simulink model "BdotControl_STAB_SUN_GRAV"  (R2019b)
settings: Solver=FixedStepAuto  StartTime=0.0  StopTime=dm.init.duration  FixedStep=fsw.init.dt  RelTol=1e-3
InitFcn:
  | clearvars;
  | % init_param_6U;
  |  init_param_6U_AW;
  | % init_param_FS_ISSorbit;
undefined symbols (not defined in the file or in its folder): dm, Earth, fsw, K_bdot, K_theta, WGS84
libraries: vrlib x4, dspmathops x3, aerolibtransform2 x2, simulink x1, aerolibgravity2 x1
settings Model: SimulationMode=accelerator  Creator=Jack-AOCS  LastModifiedBy=AndrewWang
settings DataIOCC: ReturnWorkspaceOutputs=off
settings DebuggingCC: ArithmeticOperatorsInVariantConditions=warning
settings SFSimCC: SimUseLocalCustomCode=off  CustomCodeUndefinedFunction=UseInterfaceOnly
settings RTWCC: RTWUseLocalCustomCode=off

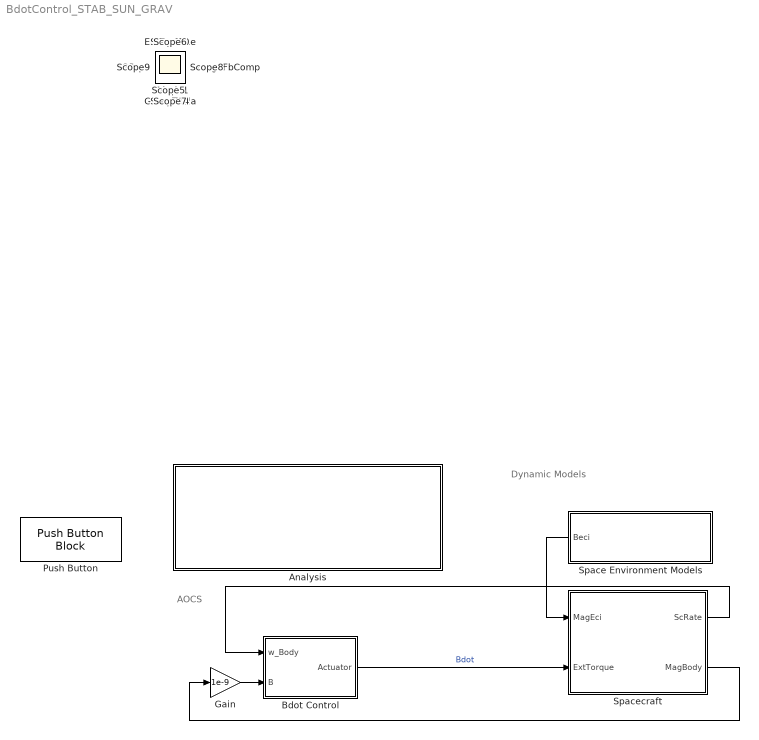
== system BdotControl_STAB_SUN_GRAV ==
  note: AOCS
  note: Dynamic Models
  Analysis : Subsystem
  Bdot Control : Subsystem
  Gain : Gain  Gain=1e-9
  Push Button : PushButtonBlock
  Space Environment Models : Subsystem
  Spacecraft : Subsystem
  BdotMc : Scope
  ExtTvsRate : Scope
  GaussTesla : Scope
  OmegaFbComp : Scope
  Rate : Scope
  Scope{,1..2,4..10,14} (11 alike) : Scope
  wires:
  Spacecraft/2(MagBody) -> Gain/1
  Space Environment Models/1(Beci) -> Spacecraft/1(MagEci)
  Bdot Control/1(Actuator) -> Spacecraft/2(ExtTorque)  "Bdot"
  Gain/1 -> Bdot Control/2(B)
  Spacecraft/1(ScRate) -> Bdot Control/1(w_Body)

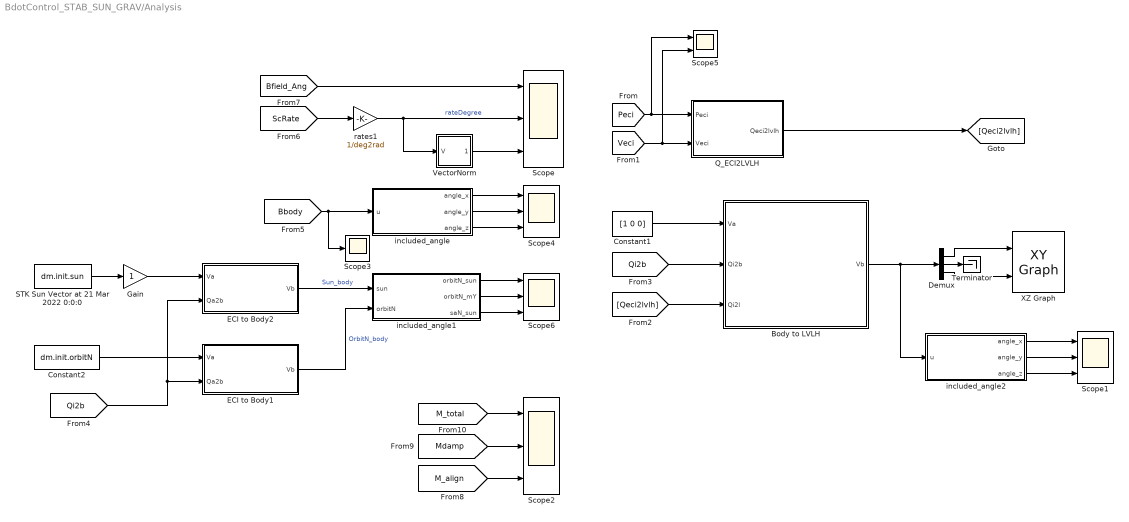
== system BdotControl_STAB_SUN_GRAV/Analysis ==
  Body to LVLH : MATLAB Function  TreatAsAtomicUnit=on
  Constant1 : Constant  Value=[1 0 0]
  Constant2 : Constant  Value=dm.init.orbitN
  Demux : Demux  Outputs=3
  ECI to Body1 : MATLAB Function  TreatAsAtomicUnit=on
  ECI to Body2 : MATLAB Function  TreatAsAtomicUnit=on
  Gain : Gain
  Q_ECI2LVLH : MATLAB Function  TreatAsAtomicUnit=on
  "STK Sun Vector at 21 Mar 2022 0:0:0 " : Constant  Value=dm.init.sun
  Scope{,1..2,4,6} (5 alike) : Scope  NumInputPorts=3
  Scope3 : Scope
  Scope5 : Scope  NumInputPorts=2
  Terminator : Terminator
  VectorNorm : Subsystem
  XZ Graph : simulink/Sinks/XY Graph  xmin=-1  xmax=1  ymin=-1  ymax=1  st=-1
  included_angle : MATLAB Function  TreatAsAtomicUnit=on
  included_angle1 : MATLAB Function  TreatAsAtomicUnit=on
  included_angle2 : MATLAB Function  TreatAsAtomicUnit=on
  rates1 : Gain  Gain=1/deg2rad
  wires:
  Q_ECI2LVLH/1(Qeci2lvlh) -> [Qeci2lvlh]
  [Peci] -> Scope5/1, Q_ECI2LVLH/1(Peci)
  Demux/1 -> XZ Graph/1
  Body to LVLH/1(Vb) -> included_angle2/1(u), Demux/1
  Constant1/1 -> Body to LVLH/1(Va)
  Demux/3 -> XZ Graph/2
  Demux/2 -> Terminator/1
  [Qeci2lvlh] -> Body to LVLH/3(Qi2l)
  [Qi2b] -> Body to LVLH/2(Qi2b)
  ECI to Body1/1(Vb) -> included_angle1/2(orbitN)  "OrbitN_body"
  "STK Sun Vector at 21 Mar 2022 0:0:0 "/1 -> Gain/1
  Gain/1 -> ECI to Body2/1(Va)
  ECI to Body2/1(Vb) -> included_angle1/1(sun)  "Sun_body"
  [Qi2b] -> ECI to Body2/2(Qa2b), ECI to Body1/2(Qa2b)
  Constant2/1 -> ECI to Body1/1(Va)
  included_angle1/2(orbitN_mY) -> Scope6/2
  included_angle1/3(saN_sun) -> Scope6/3
  included_angle1/1(orbitN_sun) -> Scope6/1
  included_angle/3(angle_z) -> Scope4/3
  included_angle/2(angle_y) -> Scope4/2
  included_angle/1(angle_x) -> Scope4/1
  [Bbody] -> Scope3/1, included_angle/1(u)
  VectorNorm/1(normV) -> Scope/3
  rates1/1 -> VectorNorm/1(V), Scope/2  "rateDegree"
  [ScRate] -> rates1/1
  included_angle2/1(angle_x) -> Scope1/1
  included_angle2/2(angle_y) -> Scope1/2
  included_angle2/3(angle_z) -> Scope1/3
  [M_total] -> Scope2/1
  [Mdamp] -> Scope2/2
  [M_align] -> Scope2/3
  [Bfield_Ang] -> Scope/1
  [Veci] -> Q_ECI2LVLH/2(Veci), Scope5/2

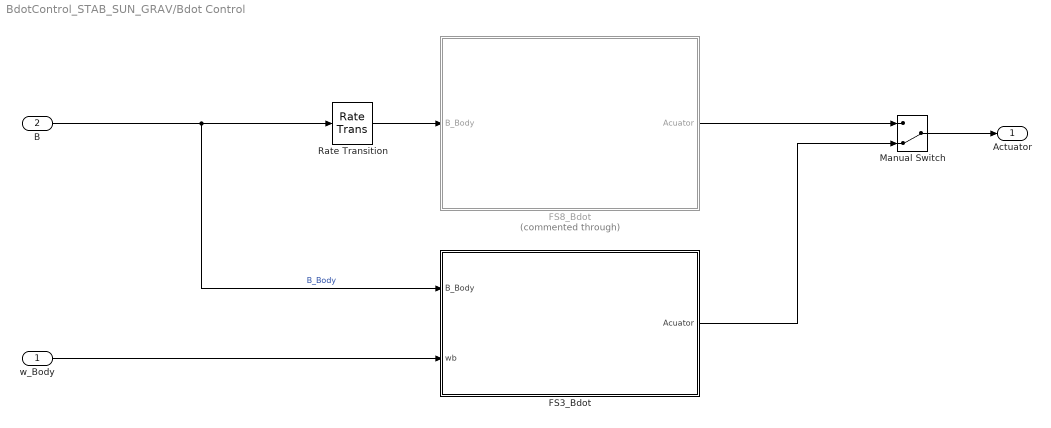
== system BdotControl_STAB_SUN_GRAV/Bdot Control ==
  w_Body : Inport
  B : Inport  Port=2
  FS3_Bdot : Subsystem
  FS8_Bdot : Subsystem  Commented=through
  Manual Switch : ManualSwitch  CurrentSetting=0
  Rate Transition : RateTransition  OutPortSampleTime=fsw.init_FS.dt
  Actuator : Outport  VectorParamsAs1DForOutWhenUnconnected=off
  wires:
  B/1 -> FS3_Bdot/1(B_Body), Rate Transition/1  "B_Body"
  Manual Switch/1 -> Actuator/1
  FS8_Bdot/1(Acuator) -> Manual Switch/1
  FS3_Bdot/1(Acuator) -> Manual Switch/2
  w_Body/1 -> FS3_Bdot/2(wb)
  Rate Transition/1 -> FS8_Bdot/1(B_Body)

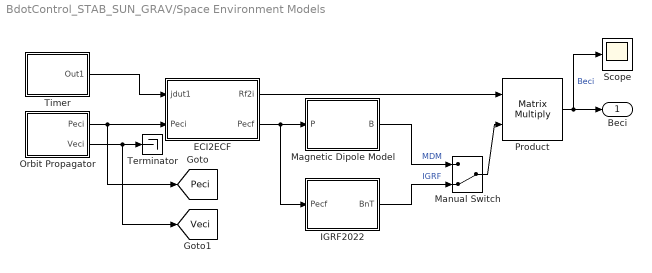
== system BdotControl_STAB_SUN_GRAV/Space Environment Models ==
  ECI2ECF : MATLAB Function  TreatAsAtomicUnit=on
  IGRF2022 : Subsystem
  Magnetic Dipole Model : MATLAB Function  TreatAsAtomicUnit=on
  Manual Switch : ManualSwitch  CurrentSetting=0
  "Orbit Propagator " : Subsystem
  Product : Product  Multiplication=Matrix(*)
  Scope : Scope
  Terminator : Terminator
  Timer : Subsystem
  Beci : Outport  VectorParamsAs1DForOutWhenUnconnected=off
  tag scope: Peci=global, Veci=global
  wires:
  ECI2ECF/1(Rf2i) -> Product/1
  Product/1 -> Scope/1, Beci/1  "Beci"
  "Orbit Propagator "/1(Peci) -> ECI2ECF/2(Peci), [Peci]
  "Orbit Propagator "/2(Veci) -> Terminator/1, [Veci]
  Timer/1(Out1) -> ECI2ECF/1(jdut1)
  ECI2ECF/2(Pecf) -> IGRF2022/1(Pecf), Magnetic Dipole Model/1(P)
  Magnetic Dipole Model/1(B) -> Manual Switch/1  "MDM"
  IGRF2022/1(BnT) -> Manual Switch/2  "IGRF"
  Manual Switch/1 -> Product/2

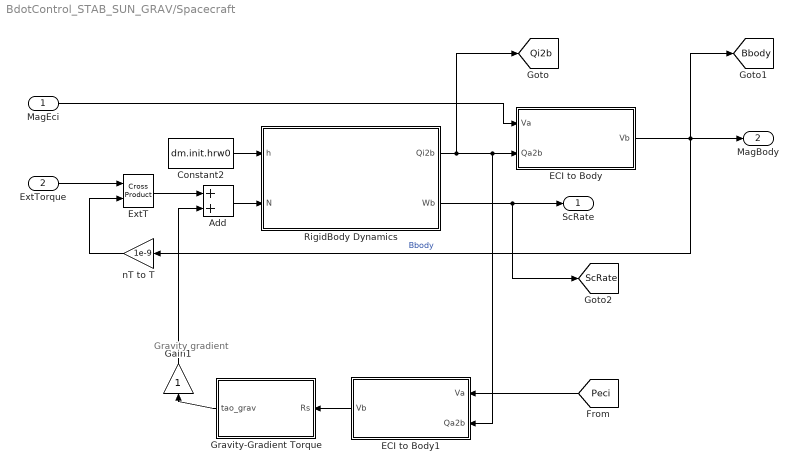
== system BdotControl_STAB_SUN_GRAV/Spacecraft ==
  note: Gravity gradient
  MagEci : Inport
  ExtTorque : Inport  Port=2
  Add : Sum
  Constant2 : Constant  Value=dm.init.hrw0
  ECI to Body : MATLAB Function  TreatAsAtomicUnit=on
  ECI to Body1 : MATLAB Function  TreatAsAtomicUnit=on
  ExtT : vrlib/Utilities/Cross Product
      settings: SourceProductBaseCode=VR
  Gain1 : Gain
  Gravity-Gradient Torque : MATLAB Function  TreatAsAtomicUnit=on
  RigidBody Dynamics : Subsystem
  nT to T : Gain  Gain=1e-9
  ScRate : Outport  VectorParamsAs1DForOutWhenUnconnected=off
  MagBody : Outport  Port=2  VectorParamsAs1DForOutWhenUnconnected=off
  tag scope: Bbody=global, Qi2b=global, ScRate=global
  wires:
  ECI to Body/1(Vb) -> [Bbody], MagBody/1, nT to T/1  "Bbody"
  RigidBody Dynamics/2(Wb) -> [ScRate], ScRate/1
  MagEci/1 -> ECI to Body/1(Va)
  RigidBody Dynamics/1(Qi2b) -> [Qi2b], ECI to Body1/2(Qa2b), ECI to Body/2(Qa2b)
  Constant2/1 -> RigidBody Dynamics/1(h)
  ExtTorque/1 -> ExtT/1
  nT to T/1 -> ExtT/2
  ExtT/1 -> Add/1
  Add/1 -> RigidBody Dynamics/2(N)
  Gravity-Gradient Torque/1(tao_grav) -> Gain1/1
  [Peci] -> ECI to Body1/1(Va)
  ECI to Body1/1(Vb) -> Gravity-Gradient Torque/1(Rs)
  Gain1/1 -> Add/2

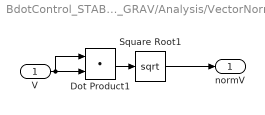
== system BdotControl_STAB_SUN_GRAV/Analysis/VectorNorm ==
  V : Inport
  Dot Product1 : DotProduct  InputSameDT=on  OutDataTypeStr=Inherit: Inherit via internal rule
  Square Root1 : Sqrt  SaturateOnIntegerOverflow=on
  normV : Outport
  wires:
  Dot Product1/1 -> Square Root1/1
  V/1 -> Dot Product1/1, Dot Product1/2
  Square Root1/1 -> normV/1

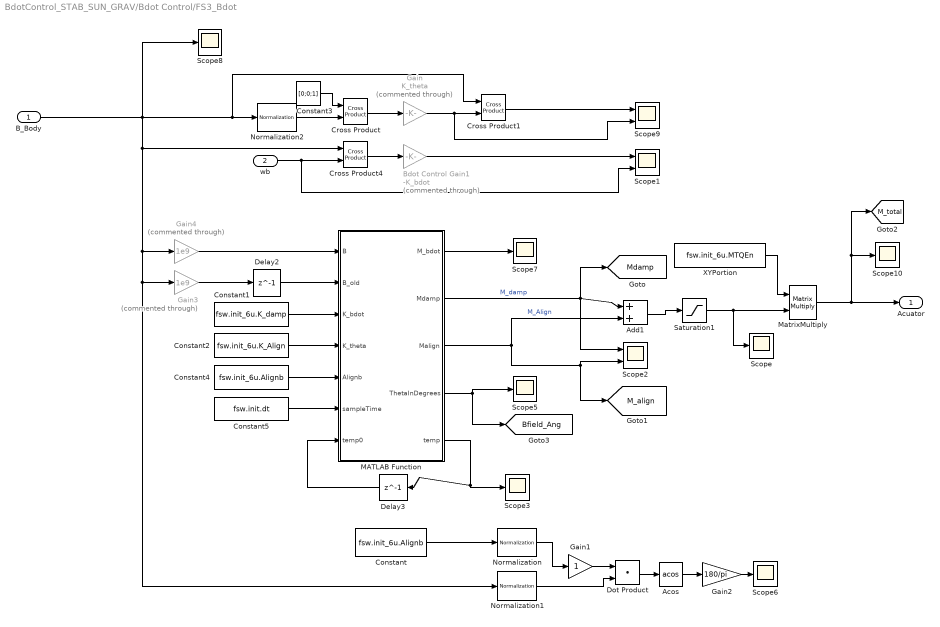
== system BdotControl_STAB_SUN_GRAV/Bdot Control/FS3_Bdot ==
  B_Body : Inport
  wb : Inport  Port=2
  Acos : Trigonometry  Operator=acos
  Add1 : Sum
  Bdot Control Gain1 : Gain  Commented=through  Gain=-K_bdot
  Constant : Constant  Value=fsw.init_6u.Alignb
  Constant1 : Constant  Value=fsw.init_6u.K_damp
  Constant2 : Constant  Value=fsw.init_6u.K_Align
  Constant3 : Constant  Value=[0;0;1]
  Constant4 : Constant  Value=fsw.init_6u.Alignb
  Constant5 : Constant  Value=fsw.init.dt
  Cross Product : vrlib/Utilities/Cross Product
      settings: SourceProductName=Simulink
  Cross Product1 : vrlib/Utilities/Cross Product
      settings: SourceProductName=Simulink
  Cross Product4 : vrlib/Utilities/Cross Product
      settings: SourceProductName=Simulink
  Delay2 : Delay  DelayLength=1  InitialCondition=[0;0;0]
  Delay3 : Delay  DelayLength=1  InitialCondition=[0;0;0]
  Dot Product : DotProduct  InputSameDT=on  OutDataTypeStr=Inherit: Inherit via internal rule
  Gain : Gain  Commented=through  Gain=K_theta
  Gain1 : Gain
  Gain2 : Gain  Gain=180/pi
  Gain3 : Gain  Commented=through  Gain=1e9
  Gain4 : Gain  Commented=through  Gain=1e9
  MATLAB Function : MATLAB Function  TreatAsAtomicUnit=on
  MatrixMultiply : Product  Multiplication=Matrix(*)
  Normalization : dspmathops/Normalization  NormType=2-norm  Bias=1e-10  NormOver=Each column  Dimension=1  roundingMode=Floor  overflowMode=off  accumDataTypeStr=Inherit: Same as product output  accumLastDataTypeStr=Inherit: Same as product output  outputDataTypeStr=Inherit: Same as product output  outputMin=[]  outputMax=[]  outputLastDataTypeStr=Inherit: Same as product output
      settings: SourceProductName=DSP System Toolbox
  Normalization1 : dspmathops/Normalization  NormType=2-norm  Bias=1e-10  NormOver=Each column  Dimension=1  roundingMode=Floor  overflowMode=off  accumDataTypeStr=Inherit: Same as product output  accumLastDataTypeStr=Inherit: Same as product output  outputDataTypeStr=Inherit: Same as product output  outputMin=[]  outputMax=[]  outputLastDataTypeStr=Inherit: Same as product output
      settings: SourceProductName=DSP System Toolbox
  Normalization2 : dspmathops/Normalization  NormType=Squared 2-norm  Bias=1e-10  NormOver=Each column  Dimension=1  roundingMode=Floor  overflowMode=off  accumDataTypeStr=Inherit: Same as product output  accumLastDataTypeStr=Inherit: Same as product output  outputDataTypeStr=Inherit: Same as product output  outputMin=[]  outputMax=[]  outputLastDataTypeStr=Inherit: Same as product output
      settings: SourceProductName=DSP System Toolbox
  Saturation1 : Saturate  UpperLimit=fsw.init_6u.MTQMax  LowerLimit=-fsw.init_6u.MTQMax
  Scope{,3,5..8,10} (7 alike) : Scope
  Scope1 : Scope  NumInputPorts=2
  Scope2 : Scope  NumInputPorts=2
  Scope9 : Scope  NumInputPorts=2
  XYPortion : Constant  Value=fsw.init_6u.MTQEn
  Acuator : Outport
  tag scope: Bfield_Ang=global, M_align=global, M_total=global, Mdamp=global
  wires:
  MATLAB Function/1(M_bdot) -> Scope7/1
  Add1/1 -> Saturation1/1
  Gain3/1 -> Delay2/1
  MatrixMultiply/1 -> [M_total], Scope10/1, Acuator/1
  Gain4/1 -> MATLAB Function/1(B)
  Cross Product1/1 -> Scope9/1
  Delay2/1 -> MATLAB Function/2(B_old)
  wb/1 -> Scope1/2, Cross Product4/2
  Bdot Control Gain1/1 -> Scope1/1
  Acos/1 -> Gain2/1
  B_Body/1 -> Scope8/1, Normalization1/1, Gain3/1, Gain4/1, Cross Product4/1, Cross Product1/1, Normalization2/1
  Normalization/1 -> Gain1/1
  MATLAB Function/5(temp) -> Scope3/1, Delay3/1
  Constant/1 -> Normalization/1
  Dot Product/1 -> Acos/1
  Saturation1/1 -> MatrixMultiply/2, Scope/1
  MATLAB Function/3(Malign) -> Add1/2, [M_align], Scope2/2  "M_Align"
  Cross Product4/1 -> Bdot Control Gain1/1
  Normalization2/1 -> Cross Product/2
  Gain2/1 -> Scope6/1
  Constant2/1 -> MATLAB Function/4(K_theta)
  Constant3/1 -> Cross Product/1
  Normalization1/1 -> Dot Product/2
  Gain/1 -> Scope9/2, Cross Product1/2
  MATLAB Function/4(ThetaInDegrees) -> Scope5/1, [Bfield_Ang]
  Delay3/1 -> MATLAB Function/7(temp0)
  Cross Product/1 -> Gain/1
  Gain1/1 -> Dot Product/1
  Constant1/1 -> MATLAB Function/3(K_bdot)
  XYPortion/1 -> MatrixMultiply/1
  MATLAB Function/2(Mdamp) -> Add1/1, [Mdamp], Scope2/1  "M_damp"
  Constant4/1 -> MATLAB Function/5(Alignb)
  Constant5/1 -> MATLAB Function/6(sampleTime)

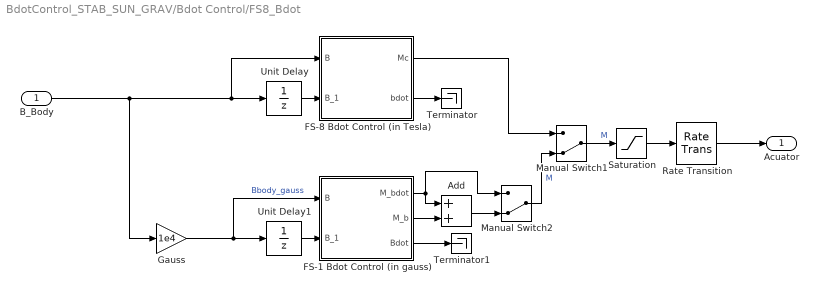
== system BdotControl_STAB_SUN_GRAV/Bdot Control/FS8_Bdot ==
  B_Body : Inport
  Add : Sum
  FS-1 Bdot Control (in gauss) : MATLAB Function  TreatAsAtomicUnit=on
  FS-8 Bdot Control (in Tesla) : MATLAB Function  TreatAsAtomicUnit=on
  Gauss : Gain  Gain=1e4
  Manual Switch1 : ManualSwitch  CurrentSetting=0
  Manual Switch2 : ManualSwitch  CurrentSetting=0
  Rate Transition : RateTransition  OutPortSampleTime=fsw.init_FS.bdot_period
  Saturation : Saturate  UpperLimit=30  LowerLimit=-30
  Terminator : Terminator
  Terminator1 : Terminator
  Unit Delay : UnitDelay  SampleTime=-1  HasFrameUpgradeWarning=on
  Unit Delay1 : UnitDelay  SampleTime=-1  HasFrameUpgradeWarning=on
  Acuator : Outport
  wires:
  B_Body/1 -> FS-8 Bdot Control (in Tesla)/1(B), Unit Delay/1, Gauss/1
  Add/1 -> Manual Switch2/2
  Unit Delay1/1 -> FS-1 Bdot Control (in gauss)/2(B_1)
  Saturation/1 -> Rate Transition/1
  FS-1 Bdot Control (in gauss)/3(Bdot) -> Terminator1/1
  FS-8 Bdot Control (in Tesla)/1(Mc) -> Manual Switch1/1
  FS-1 Bdot Control (in gauss)/2(M_b) -> Add/2
  Gauss/1 -> FS-1 Bdot Control (in gauss)/1(B), Unit Delay1/1  "Bbody_gauss"
  FS-8 Bdot Control (in Tesla)/2(bdot) -> Terminator/1
  Manual Switch2/1 -> Manual Switch1/2  "M"
  Manual Switch1/1 -> Saturation/1  "M"
  FS-1 Bdot Control (in gauss)/1(M_bdot) -> Manual Switch2/1, Add/1
  Unit Delay/1 -> FS-8 Bdot Control (in Tesla)/2(B_1)
  Rate Transition/1 -> Acuator/1

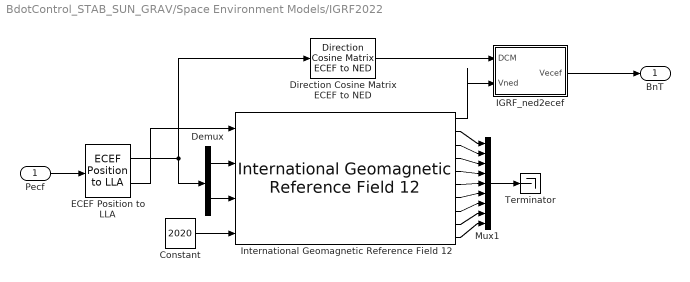
== system BdotControl_STAB_SUN_GRAV/Space Environment Models/IGRF2022 ==
  Pecf : Inport
  Constant : Constant  Value=2020
  Demux : Demux  Outputs=2
  Direction Cosine Matrix ECEF to NED : aerolibtransform2/Direction Cosine Matrix ECEF to NED
      settings: SourceProductName=Aerospace Blockset  SourceProductBaseCode=AE
  ECEF Position to LLA : aerolibtransform2/ECEF Position to LLA  units=Metric (MKS)  ptype=Earth (WGS84)  F=1/298.257223563  R=6378137
      settings: SourceProductName=Aerospace Blockset  SourceProductBaseCode=AE
  IGRF_ned2ecef : MATLAB Function  TreatAsAtomicUnit=on
  International Geomagnetic Reference Field 12 : aerolibgravity2/International Geomagnetic Reference Field 12  units=Metric (MKS)  time_in=on  month=January  day=1  year=2020  action=None  sv_out=on
      settings: SourceProductName=Aerospace Blockset  SourceProductBaseCode=AE
  Mux1 : Mux  Inputs=9
  Terminator : Terminator
  BnT : Outport  VectorParamsAs1DForOutWhenUnconnected=off
  wires:
  International Geomagnetic Reference Field 12/7 -> Mux1/6
  International Geomagnetic Reference Field 12/4 -> Mux1/3
  International Geomagnetic Reference Field 12/3 -> Mux1/2
  International Geomagnetic Reference Field 12/6 -> Mux1/5
  International Geomagnetic Reference Field 12/5 -> Mux1/4
  International Geomagnetic Reference Field 12/9 -> Mux1/8
  International Geomagnetic Reference Field 12/8 -> Mux1/7
  International Geomagnetic Reference Field 12/10 -> Mux1/9
  Pecf/1 -> ECEF Position to LLA/1
  Mux1/1 -> Terminator/1
  International Geomagnetic Reference Field 12/2 -> Mux1/1
  ECEF Position to LLA/1 -> Demux/1, Direction Cosine Matrix ECEF to NED/1
  ECEF Position to LLA/2 -> International Geomagnetic Reference Field 12/1
  Constant/1 -> International Geomagnetic Reference Field 12/4
  Demux/1 -> International Geomagnetic Reference Field 12/2
  Demux/2 -> International Geomagnetic Reference Field 12/3
  Direction Cosine Matrix ECEF to NED/1 -> IGRF_ned2ecef/1(DCM)
  IGRF_ned2ecef/1(Vecef) -> BnT/1
  International Geomagnetic Reference Field 12/1 -> IGRF_ned2ecef/2(Vned)

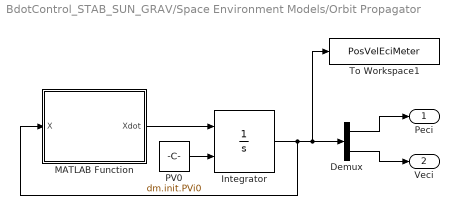
== system BdotControl_STAB_SUN_GRAV/Space Environment Models/Orbit Propagator  ==
  Demux : Demux  Outputs=2
  Integrator : Integrator  InitialConditionSource=external
  MATLAB Function : MATLAB Function  TreatAsAtomicUnit=on
  PV0 : Constant  Value=dm.init.PVi0
  To Workspace1 : ToWorkspace  VariableName=PosVelEciMeter  SaveFormat=Timeseries  SampleTime=-1
  Peci : Outport  VectorParamsAs1DForOutWhenUnconnected=off
  Veci : Outport  Port=2  VectorParamsAs1DForOutWhenUnconnected=off
  wires:
  Demux/2 -> Veci/1
  MATLAB Function/1(Xdot) -> Integrator/1
  Integrator/1 -> To Workspace1/1, Demux/1, MATLAB Function/1(X)
  Demux/1 -> Peci/1
  PV0/1 -> Integrator/2

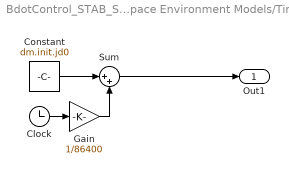
== system BdotControl_STAB_SUN_GRAV/Space Environment Models/Timer ==
  Clock : Clock
  Constant : Constant  Value=dm.init.jd0
  Gain : Gain  Gain=1/86400
  Sum : Sum  Inputs=|++
  Out1 : Outport  VectorParamsAs1DForOutWhenUnconnected=off
  wires:
  Clock/1 -> Gain/1
  Gain/1 -> Sum/2
  Constant/1 -> Sum/1
  Sum/1 -> Out1/1

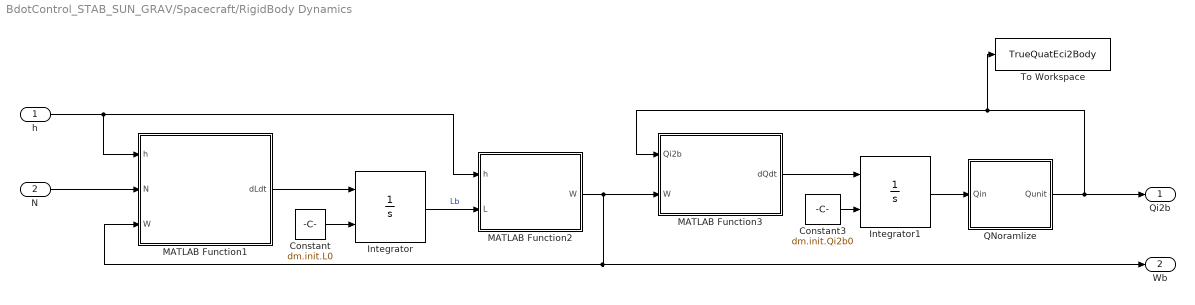
== system BdotControl_STAB_SUN_GRAV/Spacecraft/RigidBody Dynamics ==
  h : Inport
  N : Inport  Port=2
  Constant : Constant  Value=dm.init.L0
  Constant3 : Constant  Value=dm.init.Qi2b0
  Integrator : Integrator  InitialConditionSource=external
  Integrator1 : Integrator  InitialConditionSource=external
  MATLAB Function1 : MATLAB Function  TreatAsAtomicUnit=on
  MATLAB Function2 : MATLAB Function  TreatAsAtomicUnit=on
  MATLAB Function3 : MATLAB Function  TreatAsAtomicUnit=on
  QNoramlize : Subsystem
  To Workspace : ToWorkspace  VariableName=TrueQuatEci2Body  SaveFormat=Timeseries  SampleTime=-1
  Qi2b : Outport  VectorParamsAs1DForOutWhenUnconnected=off
  Wb : Outport  Port=2  VectorParamsAs1DForOutWhenUnconnected=off
  wires:
  Constant/1 -> Integrator/2
  N/1 -> MATLAB Function1/2(N)
  MATLAB Function1/1(dLdt) -> Integrator/1
  MATLAB Function3/1(dQdt) -> Integrator1/1
  Constant3/1 -> Integrator1/2
  MATLAB Function2/1(W) -> MATLAB Function3/2(W), Wb/1, MATLAB Function1/3(W)
  Integrator/1 -> MATLAB Function2/2(L)  "Lb"
  h/1 -> MATLAB Function2/1(h), MATLAB Function1/1(h)
  Integrator1/1 -> QNoramlize/1(Qin)
  QNoramlize/1(Qunit) -> Qi2b/1, To Workspace/1, MATLAB Function3/1(Qi2b)

== system BdotControl_STAB_SUN_GRAV/Spacecraft/RigidBody Dynamics/QNoramlize ==
  Qin : Inport
  Divide : Product  Inputs=*/
  VectorNorm : Subsystem
  Qunit : Outport
  wires:
  Qin/1 -> VectorNorm/1(V), Divide/1
  Divide/1 -> Qunit/1
  VectorNorm/1(normV) -> Divide/2

== system BdotControl_STAB_SUN_GRAV/Spacecraft/RigidBody Dynamics/QNoramlize/VectorNorm ==
  V : Inport
  Dot Product1 : DotProduct  InputSameDT=on  OutDataTypeStr=Inherit: Inherit via internal rule
  Square Root1 : Sqrt  SaturateOnIntegerOverflow=on
  normV : Outport
  wires:
  Dot Product1/1 -> Square Root1/1
  V/1 -> Dot Product1/2, Dot Product1/1
  Square Root1/1 -> normV/1

== matlab function BdotControl_STAB_SUN_GRAV/Bdot Control/FS8_Bdot/FS-8 Bdot Control (in Tesla) ==
  settings: updateMethod=DISCRETE
  data: B input; Mc output; B_1 input; fsw parameter; bdot output
%% Bdot Control Rev
function [Mc,bdot] = Bdot(B, B_1, fsw)

mag   = norm(B);

if mag~=0 && norm(B_1)~=0 %this is a poka-yoke
    b   =  B/norm(B);
    b_1 =  B_1/norm(B_1);
    bdot = (b-b_1)/fsw.init_FS.dt;
    sdot = (bdot-dot(b,bdot).*b)/norm(B);
    Mc = -fsw.init_FS.bdot_gain.*sdot;
else
    Mc = zeros(3,1);
    bdot =zeros(3,1);
    return;
end

== matlab function BdotControl_STAB_SUN_GRAV/Analysis/included_angle ==
  data: u input; angle_x output; angle_y output; angle_z output
function [angle_x, angle_y, angle_z]  = get_angle(u)
x = [1 0 0];
y = [0 1 0];
z = [0 0 1];
u = u/norm(u);
angle_x = acosd(dot(x,u));
angle_y = acosd(dot(y,u));
angle_z = acosd(dot(z,u));

== matlab function BdotControl_STAB_SUN_GRAV/Analysis/ECI to Body1 ==
  data: Va input; Qa2b input; Vb output
function Vb = EciToBody(Va,Qa2b)
Qb2a = QInv(Qa2b);
qout = QMul(QMul(Qb2a, [0;Va]), Qa2b);
Vb   = [qout(2) qout(3) qout(4)]';

== matlab function BdotControl_STAB_SUN_GRAV/Analysis/included_angle1 ==
  data: sun input; orbitN_sun output; orbitN_mY output; saN_sun output; orbitN input
function [orbitN_sun, orbitN_mY, saN_sun]  = get_angle(sun,orbitN)

orbitN_norm = orbitN/norm(orbitN);
sun_norm = sun/norm(sun);
orbitN_sun = acosd(dot(orbitN_norm,sun_norm));


minus_y = [0 -1 0];
orbitN_mY = acosd(dot(orbitN_norm,minus_y));

minus_z = [0 0 -1];
saN_sun = acosd(dot(sun_norm,minus_z));

== matlab function BdotControl_STAB_SUN_GRAV/Analysis/ECI to Body2 ==
  data: Va input; Qa2b input; Vb output
function Vb = EciToBody(Va,Qa2b)
Qb2a = QInv(Qa2b);
qout = QMul(QMul(Qb2a, [0;Va]), Qa2b);
Vb   = [qout(2) qout(3) qout(4)]';

== matlab function BdotControl_STAB_SUN_GRAV/Bdot Control/FS8_Bdot/FS-1 Bdot Control (in gauss) ==
  settings: updateMethod=DISCRETE
  data: B input; M_bdot output; B_1 input; fsw parameter; M_b output; Bdot output
%% Bdot Control Rev
function [M_bdot,M_b,Bdot] = Bdot(B, B_1, fsw)

mag   = norm(B);

if mag~=0 && norm(B_1)~=0 %this is a poka-yoke
    Bdot = (B-B_1)/fsw.init_FS.dt;
    M_bdot = -fsw.init_FS.bdot_gain.*Bdot;
    M_b = fsw.init_FS.b_gain.*[B(3) 0 -B(1)]';
else
    M_bdot = zeros(3,1);
    M_b = zeros(3,1);
    Bdot =zeros(3,1);
    return;
end

== matlab function BdotControl_STAB_SUN_GRAV/Analysis/Q_ECI2LVLH ==
  data: Peci input; Qeci2lvlh output; Veci input
function Qeci2lvlh = q_eci2vlh(Peci,Veci)
lvlhz = -Peci/norm(Peci);
lvlhy = -cross(Peci,Veci)/norm(cross(Peci,Veci));
lvlhx = cross(lvlhy,lvlhz);
Meci2lvlh = [lvlhx lvlhy lvlhz];
Qeci2lvlh = Mat2Q(Meci2lvlh);
mag = norm(Qeci2lvlh);
if mag~=1 && mag~=0
    Qeci2lvlh = Qeci2lvlh/mag;
%     disp('QNORM');
end

== matlab function BdotControl_STAB_SUN_GRAV/Analysis/Body to LVLH ==
  data: Va input; Qi2b input; Vb output; Qi2l input
function Vb = EciToBody(Va,Qi2b,Qi2l)
Qb2i = QInv(Qi2b);
Qb2l = QMul(Qb2i,Qi2l);

qout = QMul(QMul(QInv(Qb2l), [0;Va]), Qb2l);
Vb   = [qout(2) qout(3) qout(4)]';

== matlab function BdotControl_STAB_SUN_GRAV/Analysis/included_angle2 ==
  data: u input; angle_x output; angle_y output; angle_z output
function [angle_x, angle_y, angle_z]  = get_angle(u)
x = [1 0 0];
y = [0 1 0];
z = [0 0 1];
u = u/norm(u);
angle_x = acosd(dot(x,u));
angle_y = acosd(dot(y,u));
angle_z = acosd(dot(z,u));

== matlab function BdotControl_STAB_SUN_GRAV/Spacecraft/Gravity-Gradient Torque ==
  data: Rs input; tao_grav output; dm parameter
function tao_grav = dist_gravity(Rs, dm)

% from Wertx p567
% Rs_hat = ECI Position unit vector in body frame
Rs_hat = -Rs/norm(Rs);
tao_grav = ((3*dm.init.mu_e/norm(Rs)^3)*cross(Rs_hat, dm.init.Ib*Rs_hat));

== matlab function BdotControl_STAB_SUN_GRAV/Bdot Control/FS3_Bdot/MATLAB Function ==
  data: B input; M_bdot output; Mdamp output; B_old input; K_bdot input; K_theta input; Alignb input; sampleTime input; Malign output; ThetaInDegrees output; temp output; temp0 input
% function [Mdamp,Malign,temp,ThetaInDegrees] = fcn(B,B_old,K_bdot,K_theta,temp0)
function [M_bdot,Mdamp,Malign,ThetaInDegrees,temp] = fcn(B,B_old,K_bdot,K_theta,Alignb, sampleTime,temp0)
% % FS3 Control Therom
% temp = cross(B,B_old)/norm(B)^2;
% %加上bold = 0的防呆
% w = (temp-temp0)/epoch.sampleTime;
% temp2 = -K_bdot.*w; %add /norm(B)^2
% Mdamp = cross(B,temp2);
% Zb = [0;0;1];
% temp3 = K_theta.*cross(Zb,B./norm(B));%ori
% % temp3 = K_theta.*cross(Zb,B);
% Malign = cross(B,temp3);
% CosTheta = dot(Zb,B)/(norm(Zb)*norm(B));
% ThetaInDegrees = acosd(CosTheta);
% % b = B/norm(B);
% % bdot = (B-B_old)/epoch.sampleTime/norm(B);
% % M_bdot = -K_bdot/norm(B) .* (bdot-(dot(bdot,b)*b));

%% 6U Control Therom
if B_old~=0 & temp0 ~= 0 %加上bold = 0的防呆
   temp = cross(B,B_old)/norm(B)^2;
    w = (temp-temp0)/sampleTime;
    temp2 = -K_bdot.*w; %add /norm(B)^2
    Mdamp = cross(B,temp2);
else
    if B_old~=0
        temp = cross(B,B_old)/norm(B)^2;
    else
        temp = [0 0 0]';
    end
    Mdamp = [0 0 0]';
end
    temp3 = K_theta.*cross(Alignb,B./norm(B));%ori
    Malign = cross(B,temp3);
    CosTheta = dot(Alignb,B)/(norm(Alignb)*norm(B));
    ThetaInDegrees = acosd(CosTheta);

%% Dodo's try
b = B/norm(B);
b_old = B_old/norm(B);
bdot = (b-b_old)/sampleTime/norm(b);
% M_bdot = -K_bdot/norm(B) .* (bdot);
%% Bdot control for Forsat8
M_bdot = -K_bdot.*(bdot-(bdot.*b).*b)/norm(B);

== matlab function BdotControl_STAB_SUN_GRAV/Space Environment Models/ECI2ECF ==
  data: Rf2i output; jdut1 input; Pecf output; Peci input
%% ECI to ECEF Transformation
function [Rf2i, Pecf]  = ECI2ECF(jdut1, Peci)
Ri2f  = R3(JD2GMST(jdut1));
Pecf  = Ri2f*Peci; %in m
Rf2i  = Ri2f';

== matlab function BdotControl_STAB_SUN_GRAV/Space Environment Models/IGRF2022/IGRF_ned2ecef ==
  data: DCM input; Vecef output; Vned input
function Vecef = fcn(DCM,Vned)

Vecef = DCM'*Vned;

== matlab function BdotControl_STAB_SUN_GRAV/Space Environment Models/Magnetic Dipole Model ==
  data: P input; B output; dm parameter
function B = MagDipole(P, dm)

B = MagneticDipole(P, dm.init.mpm);

== matlab function BdotControl_STAB_SUN_GRAV/Space Environment Models/Orbit Propagator /MATLAB Function ==
  data: X input; Xdot output; dm parameter
function Xdot = TwoBodyRHS(X, dm)

r = X(1:3);
v = X(4:6);
Xdot=[v; -(dm.init.mu_e*r/norm(r)^3)];

== matlab function BdotControl_STAB_SUN_GRAV/Spacecraft/ECI to Body ==
  data: Va input; Qa2b input; Vb output
function Vb = EciToBody(Va,Qa2b)
Qb2a = QInv(Qa2b);
qout = QMul(QMul(Qb2a, [0;Va]), Qa2b);
Vb   = [qout(2) qout(3) qout(4)]';

== matlab function BdotControl_STAB_SUN_GRAV/Spacecraft/RigidBody Dynamics/MATLAB Function1 ==
  data: h input; dLdt output; N input; W input; dm parameter
%% Euler Equation
function dLdt = EulerEquation(h,N,W,dm)
L = dm.init.Ib*W + h;
dLdt = N-cross((dm.init.Ib\(L-h)),L);

== matlab function BdotControl_STAB_SUN_GRAV/Spacecraft/RigidBody Dynamics/MATLAB Function2 ==
  data: h input; W output; L input; dm parameter
%% total angular momentum of the spacecraft
function W = InvTotAngMom(h,L,dm)
W =dm.init.Ib\(L-h);

== matlab function BdotControl_STAB_SUN_GRAV/Spacecraft/RigidBody Dynamics/MATLAB Function3 ==
  data: Qi2b input; dQdt output; W input
%% Quaternion Kinematic Equation
function dQdt = QuatKinematic(Qi2b,W)
dQdt = 0.5 * (QMul(Qi2b,[0;W]));

== matlab function BdotControl_STAB_SUN_GRAV/Spacecraft/ECI to Body1 ==
  data: Va input; Qa2b input; Vb output
function Vb = EciToBody(Va,Qa2b)
Qb2a = QInv(Qa2b);
qout = QMul(QMul(Qb2a, [0;Va]), Qa2b);
Vb   = [qout(2) qout(3) qout(4)]';
